simulink model "KalmanFilter"  (R2024a)
settings: Solver=ode4  StartTime=0.0  StopTime=2831.72  FixedStep=filter_Ts  RelTol=1e-3
InitFcn:
  | loadData;
values from neighbouring files (symbols this model uses):
  filter_Ts = 0.01    [loadData.m]
  gps_sampling_time = 0.1    [loadData.m]
  imu_sampling_time = 0.01    [loadData.m]
  p_0 = diag([1e-10, 1e-10, 100, 10,  10,  10, 0.1, 0.1, 0.1, 0.005, 0.005, 0.005, 0.003, 0.003, 0.003])    [loadData.m]
  Qk = computeImuNoise(imuData100Hz, 10000)    [loadData.m]
  Rk = diag([9.07252092613911e-11,9.07204808274199e-11,0.991470480960317,0.00998692051771264,0.00989027264124697,0.0100334320982840])    [loadData.m]
  x_0 = [lon_0;lat_0;h_0;vn_0;ve_0;vd_0;phi_0;theta_0;si_0; b_accel; b_gyro]    [loadData.m]
libraries: matrix_library x1
settings Model: Creator=amir  LastModifiedBy=havaie
settings RTWCC: GPUComputeCapability=3.5

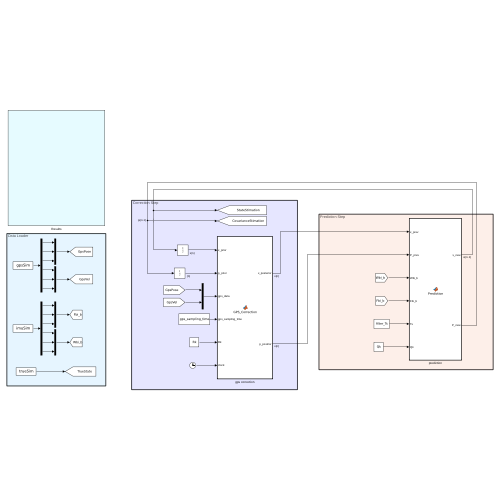
[thumbnail: Simulink's stored preview of the top-level diagram]
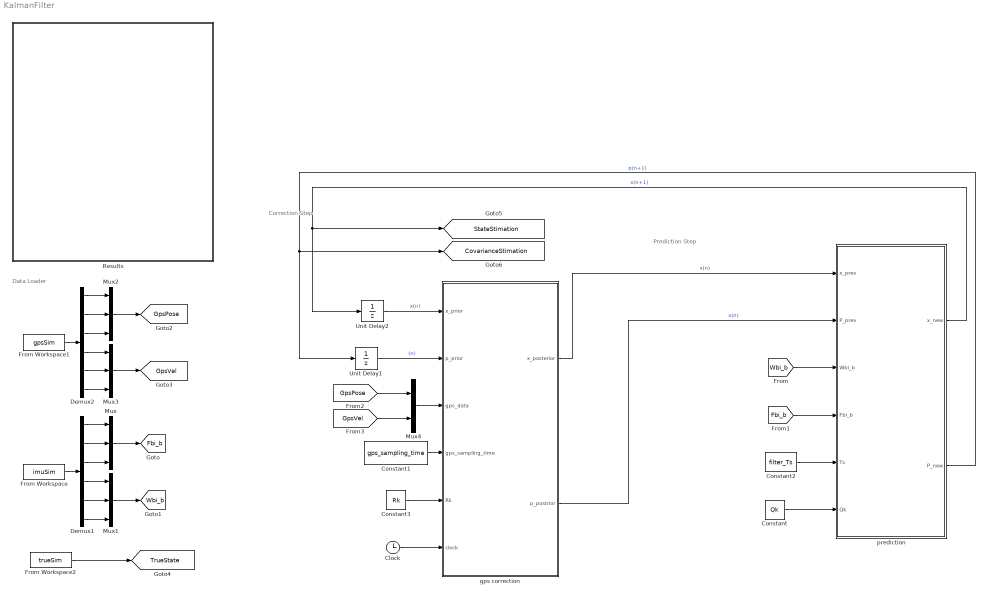
== system KalmanFilter ==
  note: Correction Step
  note: Data Loader
  note: Prediction Step
  Clock : Clock
  Constant : Constant  Value=Qk
  Constant1 : Constant  Value=gps_sampling_time
  Constant2 : Constant  Value=filter_Ts
  Constant3 : Constant  Value=Rk
  Demux1 : Demux  Outputs=6
  Demux2 : Demux  Outputs=6
  From Workspace : FromWorkspace  VariableName=imuSim  SampleTime=imu_sampling_time  Interpolate=off  OutputAfterFinalValue=Holding final value
  From Workspace1 : FromWorkspace  VariableName=gpsSim  SampleTime=gps_sampling_time  Interpolate=off  OutputAfterFinalValue=Holding final value
  From Workspace2 : FromWorkspace  VariableName=trueSim
  Mux{,1..3} (4 alike) : Mux  Inputs=3
  Mux4 : Mux  Inputs=2
  Results : Subsystem
  Unit Delay1 : UnitDelay  InitialCondition=p_0  SampleTime=-1  HasFrameUpgradeWarning=on
  Unit Delay2 : UnitDelay  InitialCondition=x_0  SampleTime=-1  HasFrameUpgradeWarning=on
  gps correction : MATLAB Function  TreatAsAtomicUnit=on
  prediction : MATLAB Function  TreatAsAtomicUnit=on
  tag scope: CovarianceStimation=global, Fbi_b=global, GpsPose=global, GpsVel=global, StateStimation=global, TrueState=global, Wbi_b=global
  wires:
  Constant2/1 -> prediction/5(Ts)
  [Fbi_b] -> prediction/4(Fbi_b)
  [Wbi_b] -> prediction/3(Wbi_b)
  From Workspace/1 -> Demux1/1
  Demux1/2 -> Mux/2
  Demux1/3 -> Mux/3
  Demux1/4 -> Mux1/1
  Demux1/5 -> Mux1/2
  Demux1/6 -> Mux1/3
  Mux/1 -> [Fbi_b]
  Mux1/1 -> [Wbi_b]
  Demux1/1 -> Mux/1
  Demux2/1 -> Mux2/1
  Demux2/5 -> Mux3/2
  Demux2/6 -> Mux3/3
  Mux2/1 -> [GpsPose]
  Mux3/1 -> [GpsVel]
  Demux2/4 -> Mux3/1
  Demux2/3 -> Mux2/3
  Demux2/2 -> Mux2/2
  Constant/1 -> prediction/6(Qk)
  Clock/1 -> gps correction/6(clock)
  Unit Delay2/1 -> gps correction/1(x_prior)  "x(n)"
  Unit Delay1/1 -> gps correction/2(p_prior)  "(n)"
  prediction/1(x_new) -> [StateStimation], Unit Delay2/1  "x(n+1)"
  prediction/2(P_new) -> [CovarianceStimation], Unit Delay1/1  "p(n+1)"
  Constant1/1 -> gps correction/4(gps_sampling_time)
  Constant3/1 -> gps correction/5(Rk)
  [GpsPose] -> Mux4/1
  [GpsVel] -> Mux4/2
  Mux4/1 -> gps correction/3(gps_data)
  From Workspace2/1 -> [TrueState]
  From Workspace1/1 -> Demux2/1
  gps correction/1(x_posterior) -> prediction/1(x_prev)  "x(n)"
  gps correction/2(p_postrior) -> prediction/2(P_prev)  "x(n)"

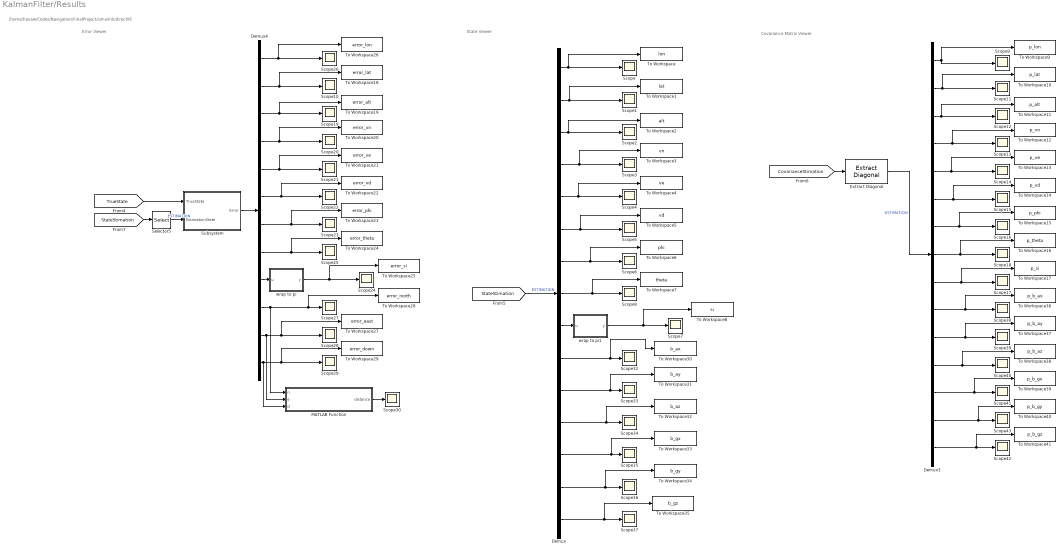
== system KalmanFilter/Results ==
  note: /home/havaie/Codes/Navigation/FinalProject/simulink/directKF
  note: Error Viewer
  note: Covariance Matrix Viewer
  note: State Viewer
  Demux : Demux  Outputs=15
  Demux3 : Demux  Outputs=15
  Demux4 : Demux  Outputs=12
  Extract Diagonal : matrix_library/Extract Diagonal
      settings: LibrarySourceBlock=|
      | simulink/Matrix
      | Operations/Extract Diagonal
  MATLAB Function : MATLAB Function  TreatAsAtomicUnit=on
  Scope{,1..30,32..43} (43 alike) : Scope
  Selector5 : Selector  InputPortWidth=15  IndexOptions=Index vector (dialog)  Indices=[1 2 3 4 5 6 7 8 9]  OutputSizes=1
  Subsystem : Subsystem
  To Workspace : ToWorkspace  VariableName=lon  SampleTime=-1
      settings: Save2DSignal=2-D array (concatenate along first dimension)
  To Workspace1 : ToWorkspace  VariableName=lat  SampleTime=-1
      settings: Save2DSignal=2-D array (concatenate along first dimension)
  To Workspace10 : ToWorkspace  VariableName=p_lat  SampleTime=-1
      settings: Save2DSignal=2-D array (concatenate along first dimension)
  To Workspace11 : ToWorkspace  VariableName=p_alt  SampleTime=-1
      settings: Save2DSignal=2-D array (concatenate along first dimension)
  To Workspace12 : ToWorkspace  VariableName=p_vn  SampleTime=-1
      settings: Save2DSignal=2-D array (concatenate along first dimension)
  To Workspace13 : ToWorkspace  VariableName=p_ve  SampleTime=-1
      settings: Save2DSignal=2-D array (concatenate along first dimension)
  To Workspace14 : ToWorkspace  VariableName=p_vd  SampleTime=-1
      settings: Save2DSignal=2-D array (concatenate along first dimension)
  To Workspace15 : ToWorkspace  VariableName=p_phi  SampleTime=-1
      settings: Save2DSignal=2-D array (concatenate along first dimension)
  To Workspace16 : ToWorkspace  VariableName=p_theta  SampleTime=-1
      settings: Save2DSignal=2-D array (concatenate along first dimension)
  To Workspace17 : ToWorkspace  VariableName=p_si  SampleTime=-1
      settings: Save2DSignal=2-D array (concatenate along first dimension)
  To Workspace18 : ToWorkspace  VariableName=error_lat  SampleTime=-1
      settings: Save2DSignal=2-D array (concatenate along first dimension)
  To Workspace19 : ToWorkspace  VariableName=error_alt  SampleTime=-1
      settings: Save2DSignal=2-D array (concatenate along first dimension)
  To Workspace2 : ToWorkspace  VariableName=alt  SampleTime=-1
      settings: Save2DSignal=2-D array (concatenate along first dimension)
  To Workspace20 : ToWorkspace  VariableName=error_vn  SampleTime=-1
      settings: Save2DSignal=2-D array (concatenate along first dimension)
  To Workspace21 : ToWorkspace  VariableName=error_ve  SampleTime=-1
      settings: Save2DSignal=2-D array (concatenate along first dimension)
  To Workspace22 : ToWorkspace  VariableName=error_vd  SampleTime=-1
      settings: Save2DSignal=2-D array (concatenate along first dimension)
  To Workspace23 : ToWorkspace  VariableName=error_phi  SampleTime=-1
      settings: Save2DSignal=2-D array (concatenate along first dimension)
  To Workspace24 : ToWorkspace  VariableName=error_theta  SampleTime=-1
      settings: Save2DSignal=2-D array (concatenate along first dimension)
  To Workspace25 : ToWorkspace  VariableName=error_si  SampleTime=-1
      settings: Save2DSignal=2-D array (concatenate along first dimension)
  To Workspace26 : ToWorkspace  VariableName=error_lon  SampleTime=-1
      settings: Save2DSignal=2-D array (concatenate along first dimension)
  To Workspace27 : ToWorkspace  VariableName=error_east  SampleTime=-1
      settings: Save2DSignal=2-D array (concatenate along first dimension)
  To Workspace28 : ToWorkspace  VariableName=error_north  SampleTime=-1
      settings: Save2DSignal=2-D array (concatenate along first dimension)
  To Workspace29 : ToWorkspace  VariableName=error_down  SampleTime=-1
      settings: Save2DSignal=2-D array (concatenate along first dimension)
  To Workspace3 : ToWorkspace  VariableName=vn  SampleTime=-1
      settings: Save2DSignal=2-D array (concatenate along first dimension)
  To Workspace30 : ToWorkspace  VariableName=b_ax  SampleTime=-1
      settings: Save2DSignal=2-D array (concatenate along first dimension)
  To Workspace31 : ToWorkspace  VariableName=b_ay  SampleTime=-1
      settings: Save2DSignal=2-D array (concatenate along first dimension)
  To Workspace32 : ToWorkspace  VariableName=b_az  SampleTime=-1
      settings: Save2DSignal=2-D array (concatenate along first dimension)
  To Workspace33 : ToWorkspace  VariableName=b_gx  SampleTime=-1
      settings: Save2DSignal=2-D array (concatenate along first dimension)
  To Workspace34 : ToWorkspace  VariableName=b_gy  SampleTime=-1
      settings: Save2DSignal=2-D array (concatenate along first dimension)
  To Workspace35 : ToWorkspace  VariableName=b_gz  SampleTime=-1
      settings: Save2DSignal=2-D array (concatenate along first dimension)
  To Workspace36 : ToWorkspace  VariableName=p_b_ax  SampleTime=-1
      settings: Save2DSignal=2-D array (concatenate along first dimension)
  To Workspace37 : ToWorkspace  VariableName=p_b_ay  SampleTime=-1
      settings: Save2DSignal=2-D array (concatenate along first dimension)
  To Workspace38 : ToWorkspace  VariableName=p_b_az  SampleTime=-1
      settings: Save2DSignal=2-D array (concatenate along first dimension)
  To Workspace39 : ToWorkspace  VariableName=p_b_gx  SampleTime=-1
      settings: Save2DSignal=2-D array (concatenate along first dimension)
  To Workspace4 : ToWorkspace  VariableName=ve  SampleTime=-1
      settings: Save2DSignal=2-D array (concatenate along first dimension)
  To Workspace40 : ToWorkspace  VariableName=p_b_gy  SampleTime=-1
      settings: Save2DSignal=2-D array (concatenate along first dimension)
  To Workspace41 : ToWorkspace  VariableName=p_b_gz  SampleTime=-1
      settings: Save2DSignal=2-D array (concatenate along first dimension)
  To Workspace5 : ToWorkspace  VariableName=vd  SampleTime=-1
      settings: Save2DSignal=2-D array (concatenate along first dimension)
  To Workspace6 : ToWorkspace  VariableName=phi  SampleTime=-1
      settings: Save2DSignal=2-D array (concatenate along first dimension)
  To Workspace7 : ToWorkspace  VariableName=theta  SampleTime=-1
      settings: Save2DSignal=2-D array (concatenate along first dimension)
  To Workspace8 : ToWorkspace  VariableName=si  SampleTime=-1
      settings: Save2DSignal=2-D array (concatenate along first dimension)
  To Workspace9 : ToWorkspace  VariableName=p_lon  SampleTime=-1
      settings: Save2DSignal=2-D array (concatenate along first dimension)
  wrap to pi : MATLAB Function  TreatAsAtomicUnit=on
  wrap to pi1 : MATLAB Function  TreatAsAtomicUnit=on
  wires:
  Demux4/2 -> To Workspace18/1, Scope10/1
  Demux3/5 -> To Workspace13/1, Scope14/1
  Demux4/1 -> To Workspace26/1, Scope26/1
  Demux/6 -> To Workspace5/1, Scope5/1
  Demux/5 -> To Workspace4/1, Scope4/1
  Demux3/3 -> To Workspace11/1, Scope12/1
  Demux3/8 -> To Workspace16/1, Scope18/1
  Demux4/4 -> To Workspace20/1, Scope20/1
  Demux/4 -> To Workspace3/1, Scope3/1
  Demux3/1 -> To Workspace9/1, Scope9/1
  Demux3/9 -> To Workspace17/1, Scope17/1
  Demux4/5 -> To Workspace21/1, Scope21/1
  Demux/1 -> To Workspace/1, Scope/1
  Demux4/3 -> To Workspace19/1, Scope19/1
  Demux3/7 -> To Workspace15/1, Scope16/1
  Demux3/6 -> To Workspace14/1, Scope15/1
  Demux4/6 -> To Workspace22/1, Scope22/1
  Demux3/4 -> To Workspace12/1, Scope13/1
  Demux/9 -> wrap to pi1/1(u)
  [CovarianceStimation] -> Extract Diagonal/1
  Demux/2 -> To Workspace1/1, Scope1/1
  Demux/3 -> To Workspace2/1, Scope2/1
  Demux3/2 -> To Workspace10/1, Scope11/1
  [TrueState] -> Subsystem/1(TrueState)
  [StateStimation] -> Selector5/1
  Subsystem/1(Error) -> Demux4/1
  Demux4/10 -> To Workspace28/1, Scope27/1, MATLAB Function/1(n)
  Demux4/11 -> MATLAB Function/2(e), To Workspace27/1, Scope28/1
  Demux4/12 -> MATLAB Function/3(d), Scope29/1, To Workspace29/1
  Demux4/7 -> To Workspace23/1, Scope23/1
  Demux4/8 -> Scope25/1, To Workspace24/1
  wrap to pi/1(y) -> Scope24/1, To Workspace25/1
  Demux/7 -> Scope6/1, To Workspace6/1
  Demux/8 -> Scope8/1, To Workspace7/1
  wrap to pi1/1(y) -> Scope7/1, To Workspace8/1
  Demux4/9 -> wrap to pi/1(u)
  [StateStimation] -> Demux/1  "ESTIMATION"
  Selector5/1 -> Subsystem/2(EstimationState)  "ESTIMATION"
  Extract Diagonal/1 -> Demux3/1  "ESTIMATION"
  Demux/10 -> To Workspace30/1, Scope32/1
  Demux/11 -> To Workspace31/1, Scope33/1
  Demux/12 -> To Workspace32/1, Scope34/1
  Demux/13 -> To Workspace33/1, Scope35/1
  Demux/14 -> To Workspace34/1, Scope36/1
  Demux/15 -> To Workspace35/1, Scope37/1
  Demux3/10 -> To Workspace36/1, Scope38/1
  Demux3/11 -> To Workspace37/1, Scope39/1
  Demux3/12 -> To Workspace38/1, Scope40/1
  Demux3/13 -> To Workspace39/1, Scope41/1
  Demux3/14 -> To Workspace40/1, Scope43/1
  Demux3/15 -> To Workspace41/1, Scope42/1
  MATLAB Function/1(distance) -> Scope30/1

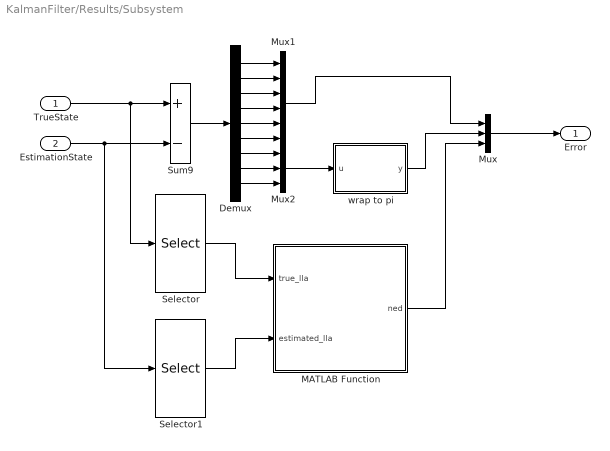
== system KalmanFilter/Results/Subsystem ==
  TrueState : Inport
  EstimationState : Inport  Port=2
  Demux : Demux  Outputs=9
  MATLAB Function : MATLAB Function  TreatAsAtomicUnit=on
  Mux : Mux  Inputs=3
  Mux1 : Mux  Inputs=6
  Mux2 : Mux  Inputs=3
  Selector : Selector  InputPortWidth=9  IndexOptions=Index vector (dialog)  Indices=[1 2 3]  OutputSizes=1
  Selector1 : Selector  InputPortWidth=9  IndexOptions=Index vector (dialog)  Indices=[1 2 3]  OutputSizes=1
  Sum9 : Sum  Inputs=+-
  wrap to pi : MATLAB Function  TreatAsAtomicUnit=on
  Error : Outport
  wires:
  TrueState/1 -> Selector/1, Sum9/1
  EstimationState/1 -> Selector1/1, Sum9/2
  Selector/1 -> MATLAB Function/1(true_lla)
  Selector1/1 -> MATLAB Function/2(estimated_lla)
  MATLAB Function/1(ned) -> Mux/3
  Mux/1 -> Error/1
  Sum9/1 -> Demux/1
  Demux/1 -> Mux1/1
  Demux/2 -> Mux1/2
  Demux/3 -> Mux1/3
  Demux/4 -> Mux1/4
  Demux/5 -> Mux1/5
  Demux/6 -> Mux1/6
  Demux/7 -> Mux2/1
  Demux/8 -> Mux2/2
  Demux/9 -> Mux2/3
  Mux1/1 -> Mux/1
  Mux2/1 -> wrap to pi/1(u)
  wrap to pi/1(y) -> Mux/2

== matlab function KalmanFilter/Results/wrap to pi1 ==
  data: u input; y output
function y = wrap_to_pi(u)
    y = mod(u + pi, 2*pi) - pi;
end

== matlab function KalmanFilter/gps correction ==
  data: x_prior input; x_posterior output; p_prior input; gps_data input; gps_sampling_time input; Rk input; p_postrior output; clock input
function [x_posterior, p_postrior]   = GPS_Correction(x_prior, p_prior, gps_data, gps_sampling_time, Rk, clock)
    % Default outputs (unchanged)
    coder.extrinsic('disp')
    x_posterior = x_prior;
    p_postrior = p_prior;
    K = zeros(15, 6);
    innovation = zeros(6, 1); 
    S = zeros(6, 6); 

    if mod(clock, gps_sampling_time) == 0 
        
        H = [eye(6), zeros(6,9)];

        innovation = gps_data - H * x_prior;
        S = H * p_prior * H' + Rk;  
        
        y_tilde = innovation;  
        K = p_prior * H' / S;  
        x_posterior = x_prior + K * y_tilde;
        I = eye(15);
        p_postrior = (I - K * H) * p_prior * (I - K * H)' + K * Rk * K';
    end
end

== matlab function KalmanFilter/prediction ==
  data: x_prev input; P_prev input; Wbi_b input; Fbi_b input; x_new output; Ts input; P_new output; Qk input
function [x_new, P_new]  = Prediction(x_prev, P_prev, Wbi_b, Fbi_b, Ts, Qk)

    dx1 = state_derivative(x_prev         , Wbi_b, Fbi_b) * Ts;
    dx2 = state_derivative(x_prev + dx1/2 , Wbi_b, Fbi_b) * Ts;
    dx3 = state_derivative(x_prev + dx2/2 , Wbi_b, Fbi_b) * Ts;
    dx4 = state_derivative(x_prev + dx3   , Wbi_b, Fbi_b) * Ts;
    
    x_new = x_prev + (dx1 + 2*dx2 + 2*dx3 + dx4)/6;

    F = Fk(x_prev, Wbi_b, Fbi_b, Ts);   
    B = Bk(x_prev, Wbi_b, Fbi_b, Ts);   
    P_new = F * P_prev * F.' + B * Qk * B.';
end

== matlab function KalmanFilter/Results/Subsystem/MATLAB Function ==
  data: true_lla input; ned output; estimated_lla input
function ned = ned_distance(true_lla, estimated_lla)
    % true_lla, estimated_lla: [lat; lon; alt] in degrees, meters
    % enu: [east; north; up] in meters
    
    % Convert to radians
    lat0 = true_lla(1);
    lon0 = true_lla(2);
    
    % Convert both to ECEF
    ref_ecef = lla_to_ecef(true_lla);
    est_ecef = lla_to_ecef(estimated_lla);
    
    % Delta vector in ECEF
    d = est_ecef - ref_ecef;

        % Rotation matrix from ECEF to ENU
    T_NE = [-sin(lat0)*cos(lon0), -sin(lat0)*sin(lon0), cos(lat0);
            -sin(lon0),           cos(lon0),            0;
             -cos(lat0)*cos(lon0),  -cos(lat0)*sin(lon0), -sin(lat0)];
    
    % Convert ECEF delta to ENU
    ned = T_NE * d;
end

function ecef = lla_to_ecef(lla)
% Convert [lat; lon; alt] to ECEF
    lat = lla(1);
    lon = lla(2);
    alt = lla(3);

    % WGS84 ellipsoid parameters
    a = 6378137.0;                % semi-major axis
    f = 1 / 298.257223563;        % flattening
    e2 = f * (2 - f);             % eccentricity squared

    sin_lat = sin(lat);
    cos_lat = cos(lat);
    sin_lon = sin(lon);
    cos_lon = cos(lon);

    N = a / sqrt(1 - e2 * sin_lat^2);  % prime vertical radius

    x = (N + alt) * cos_lat * cos_lon;
    y = (N + alt) * cos_lat * sin_lon;
    z = (N * (1 - e2) + alt) * sin_lat;

    ecef = [x; y; z];
end

== matlab function KalmanFilter/Results/Subsystem/wrap to pi ==
  data: u input; y output
function y = wrap_to_pi(u)
    y = mod(u + pi, 2*pi) - pi;
end

== matlab function KalmanFilter/Results/MATLAB Function ==
  data: n input; distance output; e input; d input
function distance = EuclidianDistance(n, e, d)
    distance = sqrt(n^2 + e^2 + d^2);
end

== matlab function KalmanFilter/Results/wrap to pi ==
  data: u input; y output
function y = wrap_to_pi(u)
    y = mod(u + pi, 2*pi) - pi;
end
